simulink model "TST_SmkLim_AirMsSel"  (R2016b)
settings: Solver=FixedStepDiscrete  StartTime=0.0  StopTime=simTime  FixedStep=sampleTime  RelTol=1e-3
values from neighbouring files (symbols this model uses):
  testCase = 1    [initTST_SmkLim_AirMsSel_001.m]    (also in initTST_SmkLim_AirMsSel_002.m = 2)
libraries: simulink x5, UnitTest_Lib x2
settings Model: Creator=zhengjinyan  LastModifiedBy=zhengjinyan
settings DebuggingCC: SignalRangeChecking=error

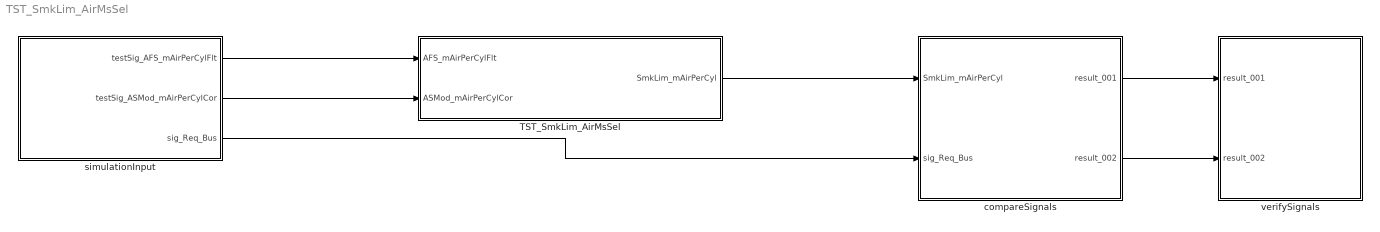
== system TST_SmkLim_AirMsSel ==
  TST_SmkLim_AirMsSel : Subsystem
  compareSignals : Subsystem
  simulationInput : Subsystem
  verifySignals : Subsystem
  wires:
  simulationInput/1(testSig_AFS_mAirPerCylFlt) -> TST_SmkLim_AirMsSel/1(AFS_mAirPerCylFlt)
  simulationInput/2(testSig_ASMod_mAirPerCylCor) -> TST_SmkLim_AirMsSel/2(ASMod_mAirPerCylCor)
  TST_SmkLim_AirMsSel/1(SmkLim_mAirPerCyl) -> compareSignals/1(SmkLim_mAirPerCyl)
  simulationInput/3(sig_Req_Bus) -> compareSignals/2(sig_Req_Bus)
  compareSignals/1(result_001) -> verifySignals/1(result_001)
  compareSignals/2(result_002) -> verifySignals/2(result_002)

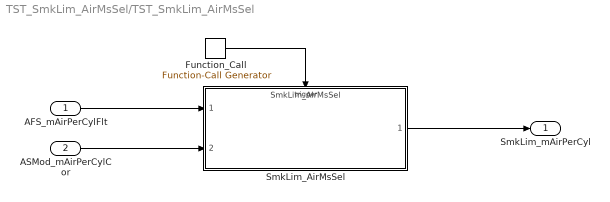
== system TST_SmkLim_AirMsSel/TST_SmkLim_AirMsSel ==
  AFS_mAirPerCylFlt : Inport
  ASMod_mAirPerCylCor : Inport  Port=2
  Function_Call : simulink/Ports & Subsystems/Function-Call Generator  sample_time=sampleTime  numberOfIterations=1
  SmkLim_AirMsSel : ModelReference  ModelNameDialog=SmkLim_AirMsSel  SimulationMode=Normal  ModelReferenceVersion=1.7  TriggerPortName=function  TriggerPortTriggerType=function-call  TriggerPortStatesWhenEnabling=held
  SmkLim_mAirPerCyl : Outport
  wires:
  Function_Call/1 -> SmkLim_AirMsSel/Trigger
  AFS_mAirPerCylFlt/1 -> SmkLim_AirMsSel/1
  ASMod_mAirPerCylCor/1 -> SmkLim_AirMsSel/2
  SmkLim_AirMsSel/1 -> SmkLim_mAirPerCyl/1

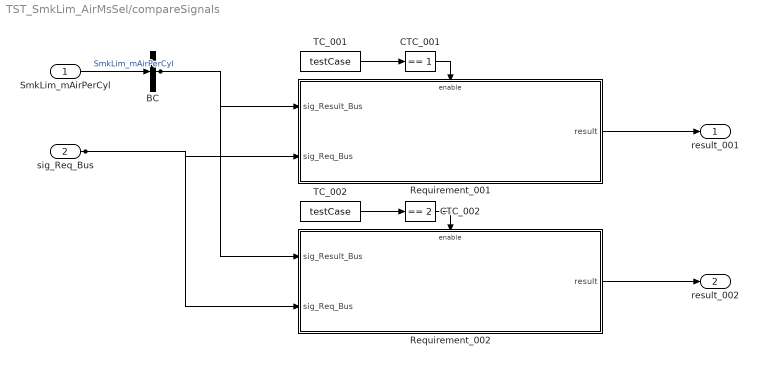
== system TST_SmkLim_AirMsSel/compareSignals ==
  SmkLim_mAirPerCyl : Inport
  sig_Req_Bus : Inport  Port=2
  BC : BusCreator  Inputs=1
  CTC_001 : simulink/Logic and Bit Operations/Compare To Constant  relop===  const=1  OutDataTypeStr=boolean
  CTC_002 : simulink/Logic and Bit Operations/Compare To Constant  relop===  const=2  OutDataTypeStr=boolean
  Requirement_001 : Subsystem
  Requirement_002 : Subsystem
  TC_001 : Constant  Value=testCase
  TC_002 : Constant  Value=testCase
  result_001 : Outport
  result_002 : Outport  Port=2
  wires:
  SmkLim_mAirPerCyl/1 -> BC/1  "SmkLim_mAirPerCyl"
  TC_001/1 -> CTC_001/1
  CTC_001/1 -> Requirement_001/Enable
  sig_Req_Bus/1 -> Requirement_001/2(sig_Req_Bus), Requirement_002/2(sig_Req_Bus)
  BC/1 -> Requirement_001/1(sig_Result_Bus), Requirement_002/1(sig_Result_Bus)
  Requirement_001/1(result) -> result_001/1
  TC_002/1 -> CTC_002/1
  CTC_002/1 -> Requirement_002/Enable
  Requirement_002/1(result) -> result_002/1

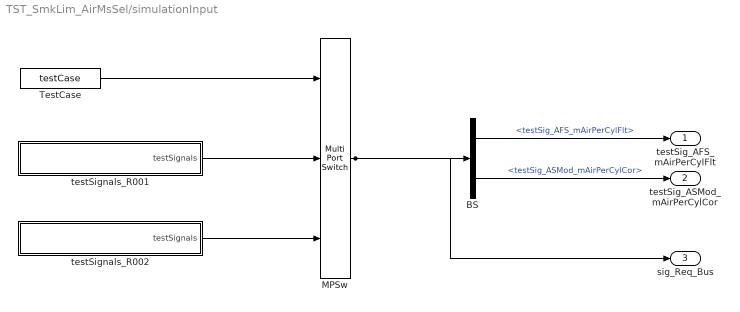
== system TST_SmkLim_AirMsSel/simulationInput ==
  BS : BusSelector  OutputSignals=testSig_AFS_mAirPerCylFlt,testSig_ASMod_mAirPerCylCor
  MPSw : MultiPortSwitch  Inputs=2  SaturateOnIntegerOverflow=on  InputSameDT=on
  TestCase : Constant  Value=testCase
  testSignals_R001 : Subsystem
  testSignals_R002 : Subsystem
  testSig_AFS_mAirPerCylFlt : Outport
  testSig_ASMod_mAirPerCylCor : Outport  Port=2
  sig_Req_Bus : Outport  Port=3
  wires:
  BS/1 -> testSig_AFS_mAirPerCylFlt/1  "<testSig_AFS_mAirPerCylFlt>"
  BS/2 -> testSig_ASMod_mAirPerCylCor/1  "<testSig_ASMod_mAirPerCylCor>"
  MPSw/1 -> BS/1, sig_Req_Bus/1
  TestCase/1 -> MPSw/1
  testSignals_R001/1(testSignals) -> MPSw/2
  testSignals_R002/1(testSignals) -> MPSw/3

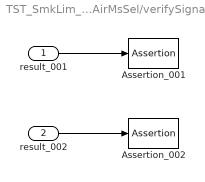
== system TST_SmkLim_AirMsSel/verifySignals ==
  result_001 : Inport
  result_002 : Inport  Port=2
  Assertion_001 : Assertion  Enabled=off
  Assertion_002 : Assertion  Enabled=off
  wires:
  result_001/1 -> Assertion_001/1
  result_002/1 -> Assertion_002/1

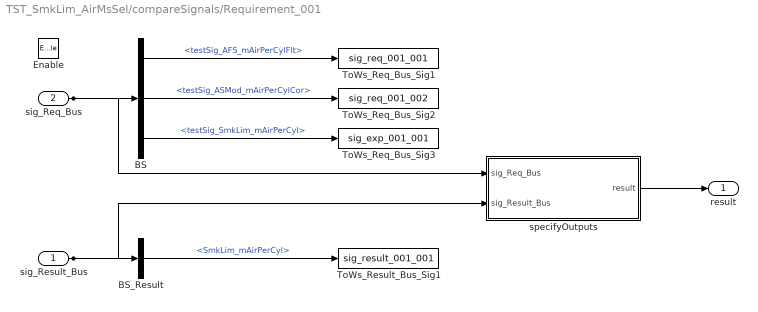
== system TST_SmkLim_AirMsSel/compareSignals/Requirement_001 ==
  sig_Result_Bus : Inport
  sig_Req_Bus : Inport  Port=2
  Enable : EnablePort
  BS : BusSelector  OutputSignals=testSig_AFS_mAirPerCylFlt,testSig_ASMod_mAirPerCylCor,testSig_SmkLim_mAirPerCyl
  BS_Result : BusSelector  OutputSignals=SmkLim_mAirPerCyl
  ToWs_Req_Bus_Sig1 : ToWorkspace  VariableName=sig_req_001_001  SaveFormat=Structure With Time
  ToWs_Req_Bus_Sig2 : ToWorkspace  VariableName=sig_req_001_002  SaveFormat=Structure With Time
  ToWs_Req_Bus_Sig3 : ToWorkspace  VariableName=sig_exp_001_001  SaveFormat=Structure With Time
  ToWs_Result_Bus_Sig1 : ToWorkspace  VariableName=sig_result_001_001  SaveFormat=Structure With Time
  specifyOutputs : Subsystem
  result : Outport
  wires:
  sig_Req_Bus/1 -> BS/1, specifyOutputs/1(sig_Req_Bus)
  BS/1 -> ToWs_Req_Bus_Sig1/1  "<testSig_AFS_mAirPerCylFlt>"
  BS/2 -> ToWs_Req_Bus_Sig2/1  "<testSig_ASMod_mAirPerCylCor>"
  BS/3 -> ToWs_Req_Bus_Sig3/1  "<testSig_SmkLim_mAirPerCyl>"
  sig_Result_Bus/1 -> BS_Result/1, specifyOutputs/2(sig_Result_Bus)
  BS_Result/1 -> ToWs_Result_Bus_Sig1/1  "<SmkLim_mAirPerCyl>"
  specifyOutputs/1(result) -> result/1

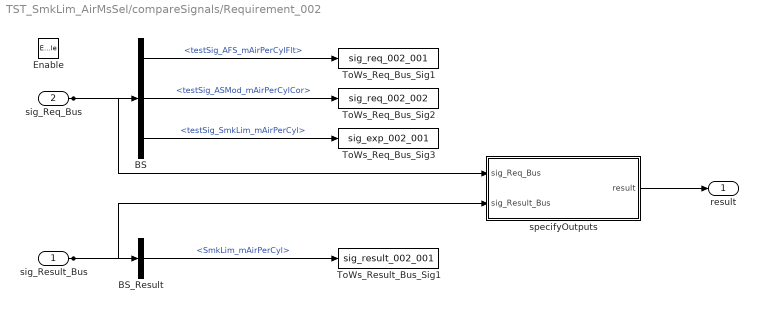
== system TST_SmkLim_AirMsSel/compareSignals/Requirement_002 ==
  sig_Result_Bus : Inport
  sig_Req_Bus : Inport  Port=2
  Enable : EnablePort
  BS : BusSelector  OutputSignals=testSig_AFS_mAirPerCylFlt,testSig_ASMod_mAirPerCylCor,testSig_SmkLim_mAirPerCyl
  BS_Result : BusSelector  OutputSignals=SmkLim_mAirPerCyl
  ToWs_Req_Bus_Sig1 : ToWorkspace  VariableName=sig_req_002_001  SaveFormat=Structure With Time
  ToWs_Req_Bus_Sig2 : ToWorkspace  VariableName=sig_req_002_002  SaveFormat=Structure With Time
  ToWs_Req_Bus_Sig3 : ToWorkspace  VariableName=sig_exp_002_001  SaveFormat=Structure With Time
  ToWs_Result_Bus_Sig1 : ToWorkspace  VariableName=sig_result_002_001  SaveFormat=Structure With Time
  specifyOutputs : Subsystem
  result : Outport
  wires:
  sig_Req_Bus/1 -> BS/1, specifyOutputs/1(sig_Req_Bus)
  BS/1 -> ToWs_Req_Bus_Sig1/1  "<testSig_AFS_mAirPerCylFlt>"
  BS/2 -> ToWs_Req_Bus_Sig2/1  "<testSig_ASMod_mAirPerCylCor>"
  BS/3 -> ToWs_Req_Bus_Sig3/1  "<testSig_SmkLim_mAirPerCyl>"
  sig_Result_Bus/1 -> BS_Result/1, specifyOutputs/2(sig_Result_Bus)
  BS_Result/1 -> ToWs_Result_Bus_Sig1/1  "<SmkLim_mAirPerCyl>"
  specifyOutputs/1(result) -> result/1

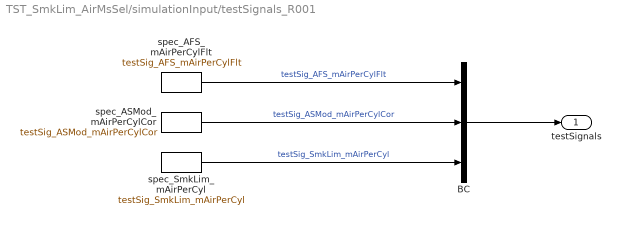
== system TST_SmkLim_AirMsSel/simulationInput/testSignals_R001 ==
  BC : BusCreator  Inputs=3
  spec_AFS_mAirPerCylFlt : FromWorkspace  VariableName=testSig_AFS_mAirPerCylFlt  Interpolate=off  OutputAfterFinalValue=Holding final value
  spec_ASMod_mAirPerCylCor : FromWorkspace  VariableName=testSig_ASMod_mAirPerCylCor  Interpolate=off  OutputAfterFinalValue=Holding final value
  spec_SmkLim_mAirPerCyl : FromWorkspace  VariableName=testSig_SmkLim_mAirPerCyl  Interpolate=off  OutputAfterFinalValue=Holding final value
  testSignals : Outport
  wires:
  BC/1 -> testSignals/1
  spec_AFS_mAirPerCylFlt/1 -> BC/1  "testSig_AFS_mAirPerCylFlt"
  spec_ASMod_mAirPerCylCor/1 -> BC/2  "testSig_ASMod_mAirPerCylCor"
  spec_SmkLim_mAirPerCyl/1 -> BC/3  "testSig_SmkLim_mAirPerCyl"

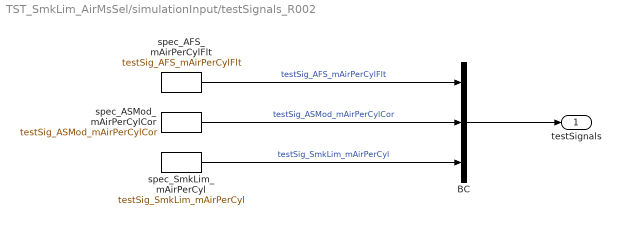
== system TST_SmkLim_AirMsSel/simulationInput/testSignals_R002 ==
  BC : BusCreator  Inputs=3
  spec_AFS_mAirPerCylFlt : FromWorkspace  VariableName=testSig_AFS_mAirPerCylFlt  Interpolate=off  OutputAfterFinalValue=Holding final value
  spec_ASMod_mAirPerCylCor : FromWorkspace  VariableName=testSig_ASMod_mAirPerCylCor  Interpolate=off  OutputAfterFinalValue=Holding final value
  spec_SmkLim_mAirPerCyl : FromWorkspace  VariableName=testSig_SmkLim_mAirPerCyl  Interpolate=off  OutputAfterFinalValue=Holding final value
  testSignals : Outport
  wires:
  BC/1 -> testSignals/1
  spec_AFS_mAirPerCylFlt/1 -> BC/1  "testSig_AFS_mAirPerCylFlt"
  spec_ASMod_mAirPerCylCor/1 -> BC/2  "testSig_ASMod_mAirPerCylCor"
  spec_SmkLim_mAirPerCyl/1 -> BC/3  "testSig_SmkLim_mAirPerCyl"

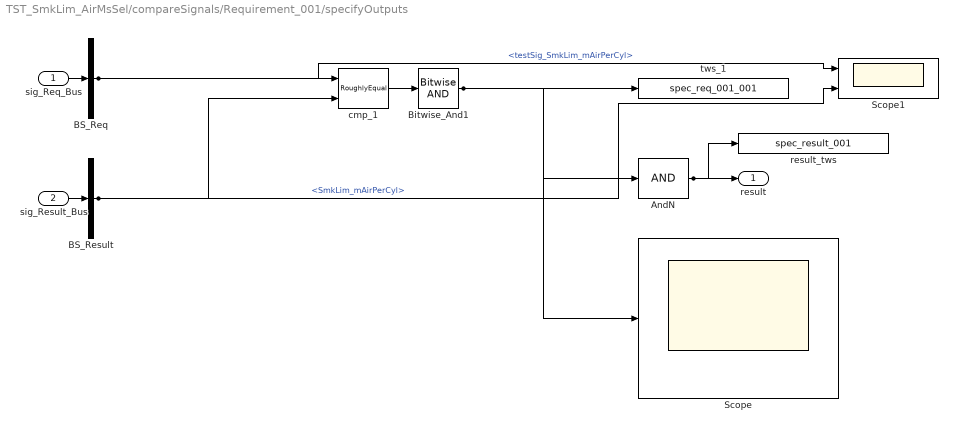
== system TST_SmkLim_AirMsSel/compareSignals/Requirement_001/specifyOutputs ==
  sig_Req_Bus : Inport
  sig_Result_Bus : Inport  Port=2
  AndN : Logic  Inputs=1
  BS_Req : BusSelector  OutputSignals=testSig_SmkLim_mAirPerCyl
  BS_Result : BusSelector  OutputSignals=SmkLim_mAirPerCyl
  Bitwise_And1 : simulink/Logic and Bit Operations/Bitwise Operator  logicop=AND  UseBitMask=off  BitMask=bin2dec('11011001')  BitMaskRealWorld=Stored Integer
  Scope : Scope
  Scope1 : Scope  NumInputPorts=2
  cmp_1 : UnitTest_Lib/RoughlyEqual  slope=0.1
  result_tws : ToWorkspace  VariableName=spec_result_001
  tws_1 : ToWorkspace  VariableName=spec_req_001_001
  result : Outport
  wires:
  sig_Req_Bus/1 -> BS_Req/1
  sig_Result_Bus/1 -> BS_Result/1
  AndN/1 -> result/1, result_tws/1
  BS_Req/1 -> cmp_1/1, Scope1/1  "<testSig_SmkLim_mAirPerCyl>"
  BS_Result/1 -> cmp_1/2, Scope1/2  "<SmkLim_mAirPerCyl>"
  cmp_1/1 -> Bitwise_And1/1
  Bitwise_And1/1 -> tws_1/1, AndN/1, Scope/1

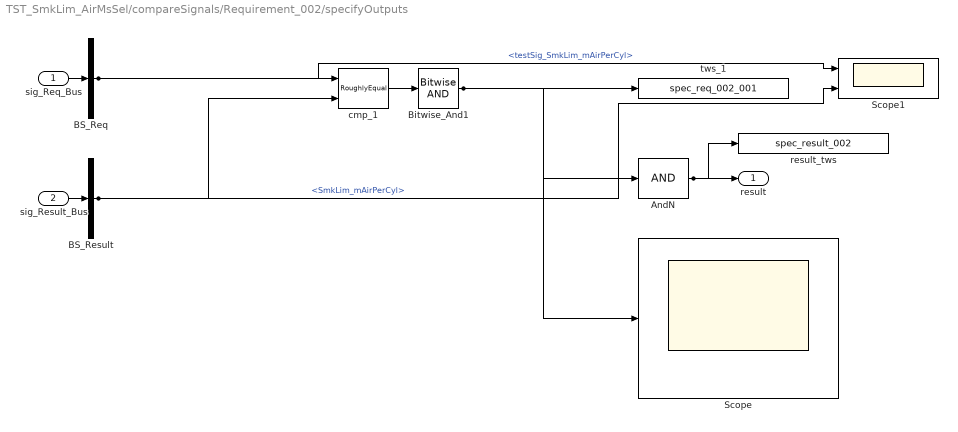
== system TST_SmkLim_AirMsSel/compareSignals/Requirement_002/specifyOutputs ==
  sig_Req_Bus : Inport
  sig_Result_Bus : Inport  Port=2
  AndN : Logic  Inputs=1
  BS_Req : BusSelector  OutputSignals=testSig_SmkLim_mAirPerCyl
  BS_Result : BusSelector  OutputSignals=SmkLim_mAirPerCyl
  Bitwise_And1 : simulink/Logic and Bit Operations/Bitwise Operator  logicop=AND  UseBitMask=off  BitMask=bin2dec('11011001')  BitMaskRealWorld=Stored Integer
  Scope : Scope
  Scope1 : Scope  NumInputPorts=2
  cmp_1 : UnitTest_Lib/RoughlyEqual  slope=0.1
  result_tws : ToWorkspace  VariableName=spec_result_002
  tws_1 : ToWorkspace  VariableName=spec_req_002_001
  result : Outport
  wires:
  sig_Req_Bus/1 -> BS_Req/1
  sig_Result_Bus/1 -> BS_Result/1
  AndN/1 -> result/1, result_tws/1
  BS_Req/1 -> cmp_1/1, Scope1/1  "<testSig_SmkLim_mAirPerCyl>"
  BS_Result/1 -> cmp_1/2, Scope1/2  "<SmkLim_mAirPerCyl>"
  cmp_1/1 -> Bitwise_And1/1
  Bitwise_And1/1 -> tws_1/1, AndN/1, Scope/1
